simulink model "tempModel_heater_Coffee_agg2"  (Simulink 10.0)
settings: Solver=ode5  StartTime=0.0  StopTime=3600  FixedStep=fixedStep  MaxStep=0.2  RelTol=1e-3
values from neighbouring files (symbols this model uses):
  maxT = 80    [ACInit.m]    (also in heater2Init.m = 82)
  minT = 70    [ACInit.m]    (also in heater2Init.m)
  Tdelta = -0.6/60    (= -0.01)    [ACInit.m]    (also in heater2Init.m = 0.0075)
undefined symbols (not defined in the file or in its folder): fixedStep, initT, startHeater
settings Model: Creator=lixuansong  LastModifiedBy=lixuansong
settings DataIOCC: SaveFormat=Dataset  ReturnWorkspaceOutputs=on
settings OptimizationCC: LifeSpan=auto
settings DebuggingCC: UnderspecifiedInitializationDetection=Simplified  MergeDetectMultiDrivingBlocksExec=error  SFUnexpectedBacktrackingDiag=error  SFNoUnconditionalDefaultTransitionDiag=error  SFExecutionAtInitializationDiag=warning  ArithmeticOperatorsInVariantConditions=error
settings HardwareCC: ProdBitPerPointer=64  ProdBitPerSizeT=64  ProdBitPerPtrDiffT=64  ProdLargestAtomicFloat=Float  ProdIntDivRoundTo=Zero  ProdEndianess=LittleEndian  ProdWordSize=64  ProdHWDeviceType=Intel->x86-64 (Windows64)
settings ModelReferenceCC: PropagateSignalLabelsOutOfModel=on
settings SFSimCC: SimUseLocalCustomCode=on  CustomCodeUndefinedFunction=FilterOut
settings RTWCC: RTWUseLocalCustomCode=on
settings CodeAppCC: StateflowObjectComments=off
settings GRTTargetCC: TargetLangStandard=C99 (ISO)  CombineOutputUpdateFcns=on  GRTInterface=off
settings ConfigComp: CovMetricSettings=dwe  CovHtmlReporting=off  CovSaveCumulativeToWorkspaceVar=off  CovSaveSingleToWorkspaceVar=off

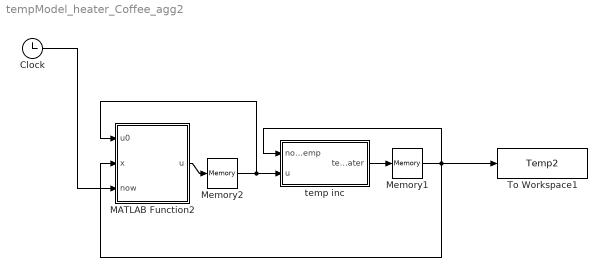
== system tempModel_heater_Coffee_agg2 ==
  Clock : Clock
  MATLAB Function2 : MATLAB Function  TreatAsAtomicUnit=on
  Memory1 : Memory  InitialCondition=initT
  Memory2 : Memory
  To Workspace1 : ToWorkspace  VariableName=Temp2  SampleTime=-1
  temp inc : MATLAB Function  TreatAsAtomicUnit=on
  wires:
  MATLAB Function2/1(u) -> Memory2/1
  Memory2/1 -> temp inc/2(u), MATLAB Function2/1(u0)
  Clock/1 -> MATLAB Function2/3(now)
  Memory1/1 -> MATLAB Function2/2(x), temp inc/1(nowTemp), To Workspace1/1
  temp inc/1(tempHeater) -> Memory1/1

== matlab function temp inc ==
  data: tempHeater output double; Tdelta parameter double; nowTemp input double; u input double; fixedStep parameter double
function tempHeater = calcTemp(Tdelta, nowTemp, u,fixedStep)

td=Tdelta*fixedStep;

tempHeater=nowTemp+u*td;


end

== matlab function MATLAB Function2 ==
  data: u0 input double; x input double; u output double; minT parameter double; maxT parameter double; startHeater parameter double; now input double; fixedStep parameter double
function u = controlHeater(u0,x, minT, maxT,startHeater,now,fixedStep)


if fix(now/fixedStep)==fix(startHeater/fixedStep)
    u=1;
elseif x<minT  && u0==0
    u=1;
elseif x>maxT && u0==1
    u=0;
else 
    u=u0;
end
